simulink model "VehicleSilSimulation"  (R2026a)
settings: configuration reference "standardSILConfigurationParams" (kept outside this file)
StopFcn:
  | fid = fopen('C:\Users\Edison Altamirano\SITLV2\AnelloSummer\optimAeroPX4SIL\HILDiagnostics\logs\session_gtfix1\matlab_error_capture.txt','a'); fprintf(fid, '--- StopFcn fired at %s ---\n', datestr(now)); [m,i] = lasterr(); fprintf(fid, 'lasterr: %s (id: %s)\n', m, i); try; le = lasterror(); fprintf(fid, 'stack:\n'); for k=1:numel(le.stack); fprintf(fid, '  %s line %d\n', le.stack(k).name, le.stack(k).line); end; catch; end; fclose(fid);
values from neighbouring files (symbols this model uses):
  CONTROLLER_RUNTIME = 1    [initVehicleSIL.m]
  stepSize_s = 0.004    [initVehicleSIL.m]
  vehicleParams = evalin('base', 'vehicleParams')    [testVehicleSIL.m]
undefined symbols (not defined in the file or in its folder): actuatorDelay_s, controllerArmed, EngineCommandBus, gpsFreq, heartbeatFreq, opts, Payload, plantSampleTime_s, referenceLatitude_deg, referenceLongitude_deg, SampleTime, ServosCommandBus
libraries: uavmavlinklib x8, simulink x8, instrumentlib x6, flightGearInterfaceLibrary x6, aerolibfltsims x3, sharedtransform x3, px4MAVLinkBridgelib x2, aerolibanimutils x1, hdlsllib x1, dspnetwork x1, robotcorelib x1, uavutilslib x1
(part 3 of 3)

== matlab function VehicleSilSimulation/vehicleSimulation/plant/f22JSBSim/packF22JSBSimInputs ==
  data: posAileron_rad input; jsbsimInputs output; posElevator_rad input; posRudder_rad input; cmdThrottle_unit input; simTime_s input; isVehicleAirborne input; controllerArmed input
function jsbsimInputs = packF22JSBSimInputs(posAileron_rad, posElevator_rad, posRudder_rad, cmdThrottle_unit, simTime_s, isVehicleAirborne, controllerArmed)
%#codegen
% Re-normalizes actuatorsF22JSBSim.slx's achieved (rate-limited) surface positions back to
% JSBSim's fcs/*-cmd-norm convention, using the same real deflection limits as
% setUpActuators.m's "f22jsbsim" case (sourced from f22.xml <flight_control> aerosurface_scale
% ranges: aileron +-0.436 rad/24.98 deg, elevator +-0.5236 rad/30 deg, rudder +-0.5236 rad/30 deg
% -- confirmed by direct grep of aircraft/f22/f22.xml's "Lateral"/"Pitch" channels, see
% PLAN_JSBSIM_SFUNCTION_F22_C130.md Phase A). Throttle is broadcast to both F119-PW-100 engine
% indices -- PX4's MAV_TYPE 1 airframe has only one throttle channel, no independent per-engine
% control in this pass. Output order matches f22JSBSim_io.xml <input> order exactly: aileron,
% elevator, rudder, throttle (bare, engine 0), throttle[1] (engine 1), gear-cmd-norm,
% left-brake-cmd-norm, right-brake-cmd-norm -- do not reorder without updating that file.
%
% PARKING BRAKE / GROUND-ROLL INTERLOCK (added 2026-08-01, PLAN_JSBSIM_SFUNCTION_F22_C130.md
% section 17): f22run-guarded (session_gtfix1) found the plant rolling and accelerating
% completely unsupervised for the ENTIRE ~178s PX4 spends on EKF-alignment/arm retries before
% this vehicle's first "armed" event -- idle turbine thrust (~1300 lbf/engine once the engine-IC
% transient below settles) with no brake command ever wired and only rolling_friction=0.02 lets
% the aircraft reach 32+ m/s before PX4 ever takes control, which is what actually corrupted the
% land-detector/TECS/runway-takeoff state machine downstream (not a sensor bug, not a JSBSim aero
% bug). Fix: hold full parking brake (both fcs/left-brake-cmd-norm and fcs/right-brake-cmd-norm
% at 1.0) AND force commanded throttle to 0 (a second, independent interlock -- this does not
% eliminate turbine idle thrust by itself, brakes carry that load) whenever controllerArmed is
% false. controllerArmed is threaded in from PX4 Interface's own existing (previously
% subsystem-local) "controllerArmed" Goto tag, now exposed as a real port -- see
% VehicleSilSimulation.slx/PX4 Interface and the plant/vehicleSimulation port chain.
%
% RELEASE CONDITION: PX4 Interface does not expose vehicle_status.nav_state or
% vehicle_attitude_setpoint over the HIL link this SIL uses (pixhawk_sil_connector is a
% source-unavailable binary S-Function whose output vector carries mapped servo/actuator values,
% not internal PX4 topics) -- true "active mode is takeoff/mission" and "valid takeoff attitude
% setpoint exists" checks from the user's original spec are therefore not directly observable in
% Simulink. Pragmatic, documented substitute: release once controllerArmed is true AND commanded
% throttle (BEFORE this function's own zero-while-disarmed override, i.e. the raw
% cmdThrottle_unit input) exceeds a small threshold -- PX4 only commands real throttle once it is
% actually trying to taxi/take off, so this approximates "a real takeoff/mission setpoint is
% driving the vehicle" using signals that actually exist here. Debounced 0.75s (persistent sample
% counter at this model's Ts, matches stepSize_s=0.004s/250Hz) before brakes actually release, per
% the user's 0.5-1s debounce request.
releaseThrottleThreshold_unit = 0.05;
debounceTime_s = 0.75;
Ts_s = 0.004;
debounceSamples = round(debounceTime_s / Ts_s);

% ONE-WAY LATCH (added after session_gtfix3, PLAN_JSBSIM_SFUNCTION_F22_C130.md section 18):
% gtfix3's LateralDebug log caught the exact mechanism -- without a latch, brakesReleased was
% recomputed fresh every step from releaseConditionCounter, which resets to 0 on the very next
% sample where cmdThrottle_unit dips at/below the threshold (release requires 0.75s sustained,
% but re-engage was a single-sample trip, no debounce in that direction). PX4 cut throttle to
% ~0 right at rotation (t=25.0-25.27s), which snapped full parking brake back on
% (fcs/left-brake-cmd-norm=fcs/right-brake-cmd-norm=1) for t=25.268-27.936s -- spanning the exact
% moment the aircraft actually left the ground (altitude climbing from t~26s onward, gear still
% commanded down). Reapplying full brake torque during that ground/air transition, when left/right
% main gear compression is momentarily asymmetric, injected a differential drag moment that seeded
% the roll/yaw divergence observed starting t=27.0-27.5s (fcs/aileron-cmd-norm and moments/l-aero-
% lbsft both diverging sharply, well before gear/gear-pos-norm even started retracting at t=28.0).
% Plant-only sign test (f22_lateral_probe.xml) had already cleared aileron/rudder sign and
% aero-derivative defects, and gear-pos-norm stayed at 1.000 through the divergence onset in both
% this run and the earlier session_gtfix2, ruling out the gear-retraction kinematic snap itself as
% the trigger -- it's specifically the brake re-engagement. Fix: once brakes have legitimately
% released (throttle sustained above threshold for the full debounce while armed), never re-engage
% for the rest of the flight -- same one-way latch pattern as gearRetracted below. A real parking
% brake wouldn't be stomped back on mid-rotation just because throttle blipped low for a moment.
persistent releaseConditionCounter brakesEverReleased
if isempty(releaseConditionCounter)
    releaseConditionCounter = int32(0);
end
if isempty(brakesEverReleased)
    brakesEverReleased = false;
end
releaseConditionNow = controllerArmed && (cmdThrottle_unit > releaseThrottleThreshold_unit);
if releaseConditionNow
    releaseConditionCounter = min(releaseConditionCounter + 1, debounceSamples);
else
    releaseConditionCounter = int32(0);
end
if ~brakesEverReleased && releaseConditionCounter >= debounceSamples
    brakesEverReleased = true;
end
brakesReleased = brakesEverReleased;

if ~controllerArmed
    cmdThrottle_unit = 0;
end
%
% gear-cmd-norm retracts once BOTH isVehicleAirborne (Memory-delayed h-agl-ft feedback from
% unpackF22JSBSimOutputs.m) is true AND simTime_s (Clock feedback) exceeds a 5s safety floor -- see
% PLAN_JSBSIM_SFUNCTION_F22_C130.md section 12 for the full history of why this specific condition
% was chosen; short version: f22.xml's "Pitch" channel has a "fcs/gear-down-q-limit" switch that
% caps commanded pitch-rate authority to 30% of normal while gear/gear-pos-norm > 0, and this
% airframe is documented as "10% unstable at subsonic" -- 30% authority alone was confirmed
% (f22run9: softened PX4 demand gains, gear permanently down, NO transition at all) to be
% insufficient for genuine STABILITY, not merely a demand/tracking mismatch -- the aircraft
% diverged into the same uncontrolled nose-up pitch runaway regardless of how gently PX4 asked for
% pitch rate. This rules out "PX4 demanding too much" as the sole cause and means gear MUST
% eventually retract to reach the full authority this airframe's own FCS was designed around.
% Earlier attempts at retraction alone (f22run6/f22run7/f22run8) each hit a different problem
% (spurious premature retraction at t=0; retraction while still parked/unarmed; a violent
% integrator-windup-release snap at the 30%->100% step transition after 22+ seconds of
% authority-limited flight) -- this version combines dynamic retraction with the SAME softened
% FW_P_RMAX_POS/FW_T_CLMB_R_SP/FW_P_LIM_MAX demand gains from the f22run9 attempt, so that
% whatever time is spent in the 30%-limited regime before liftoff accumulates much less
% integrator windup than the original unsoftened gains did, minimizing the severity of the
% eventual authority-restoration transition rather than eliminating the need for it.
%
% gearRetracted LATCH (added after f22run10): isVehicleAirborne is a raw instantaneous h-agl-ft>0.1m
% threshold (see unpackF22JSBSimOutputs.m), only delayed by a single step through the Memory block --
% NOT debounced. f22run10's groundtruth (vehicle_local_position_groundtruth in the resulting .ulg)
% showed the aircraft sitting still until simTime_s crossed 5s, then bouncing violently (z
% oscillating ~0.7-1.6m, vz swinging +-3 m/s) for ~17s before finally launching uncontrolled -- the
% bounce onset lines up exactly with the 5s floor arming the retract condition. Root cause: with
% zero gear-traverse-time (the same C130 lesson applied proactively in f22.xml), any ground-contact
% bounce that nudges h-agl-ft back and forth across the 0.1m threshold makes isVehicleAirborne (and
% therefore gearCmd_norm) chatter every step; gear position then snaps instantly on every chatter,
% injecting a contact-force impulse each time -- a resonant feedback loop that eventually threw the
% aircraft airborne rather than letting it settle. Fix: gear retraction is now a one-way persistent
% latch -- once the airborne+5s condition is true for a single step, gearRetracted stays true.
% A separate landing-extension latch below may subsequently command the gear down, but never lets
% it chatter back up after touchdown. This eliminates the takeoff chatter without
% reintroducing either of the f22run6/f22run7 premature-retraction regressions, since the latch only
% ever transitions 0->1, never back.
maxAilDefl_rad = 0.436;
maxElevatorDefl_rad = 0.5236;
maxRudderDefl_rad = 0.5236;

aileronCmd_norm = max(min(posAileron_rad / maxAilDefl_rad, 1), -1);
elevatorCmd_norm = max(min(posElevator_rad / maxElevatorDefl_rad, 1), -1);
rudderCmd_norm = max(min(posRudder_rad / maxRudderDefl_rad, 1), -1);
throttleCmd_norm = max(min(cmdThrottle_unit, 1), 0);

persistent gearRetracted gearExtendedForLanding
if isempty(gearRetracted)
    gearRetracted = false;
end
if isempty(gearExtendedForLanding)
    gearExtendedForLanding = false;
end
if ~gearRetracted && isVehicleAirborne && simTime_s > 5
    gearRetracted = true;
end
% Once a real flight has retracted the gear, the next low-AGL/contact
% indication is the only unambiguous landing cue available through this SIL
% interface. Latch the gear down at that point. The F-22 JSBSim gear has
% zero traverse time, so restoring contact geometry on this first sample
% prevents the aircraft from falling through the terrain during RTL. The
% latch also prevents the old gear chatter if the aircraft bounces.
if gearRetracted && ~gearExtendedForLanding && ~isVehicleAirborne
    gearExtendedForLanding = true;
end
gearCmd_norm = double(~gearRetracted || gearExtendedForLanding);

% Reapply symmetric wheel braking only after the landing-extension latch has
% observed the first post-flight ground contact.  brakesEverReleased must
% remain one-way during takeoff (see above), but leaving both brakes at zero
% forever made the F-22 roll/bounce beyond the 1000 s mission horizon after a
% valid NAV_LAND touchdown.  The landing latch is unavailable until the gear
% has first retracted in real flight, so this cannot reintroduce parking-brake
% chatter during rotation.  Symmetric commands also avoid a yaw impulse.
landingBrakeApplied = gearExtendedForLanding;
if ~brakesReleased || landingBrakeApplied
    leftBrakeCmd_norm = 1;
    rightBrakeCmd_norm = 1;
else
    leftBrakeCmd_norm = 0;
    rightBrakeCmd_norm = 0;
end

jsbsimInputs = [aileronCmd_norm; elevatorCmd_norm; rudderCmd_norm; ...
                throttleCmd_norm; throttleCmd_norm; ...
                gearCmd_norm; leftBrakeCmd_norm; rightBrakeCmd_norm];
end

== matlab function VehicleSilSimulation/vehicleSimulation/plant/f22JSBSim/unpackF22JSBSimOutputs ==
  data: jsbsimState input; aircraftVelInNED_mps output; jsbsimAero input; gravityScalar_mps2 input; referenceLatitude_deg input; referenceLongitude_deg input; aircraftPosInNED_m output; aircraftEulerAngles_rad output; aircraftVelInBody_mps output; aircraftAngVelInBody_radps output; aircraftAngAccelInBody_radps2 output; aircraftAccelInBody_mps2 output; DCM_be output; aircraftAccelbe_mps2 output; airspeedInBody_mps output; alpha_rad output; beta_rad output; isVehicleAirborne output
function [aircraftVelInNED_mps, aircraftPosInNED_m, aircraftEulerAngles_rad, ...
          aircraftVelInBody_mps, aircraftAngVelInBody_radps, aircraftAngAccelInBody_radps2, ...
          aircraftAccelInBody_mps2, DCM_be, aircraftAccelbe_mps2, ...
          airspeedInBody_mps, alpha_rad, beta_rad, isVehicleAirborne] = ...
          unpackF22JSBSimOutputs(jsbsimState, jsbsimAero, gravityScalar_mps2, ...
          referenceLatitude_deg, referenceLongitude_deg) %#codegen
% Converts JSBSim_SFunction's raw English-unit "State"/"Aero" output vectors (see
% f22JSBSim_io.xml for the exact property order this function assumes) into the SI
% BodyStateBus/AirDataBus fields the rest of this SIL expects. Same conversions as
% c172pJSBSim's/c130JSBSim's own unpack*JSBSimOutputs.m (aircraft-independent physics -- see
% PLAN_JSBSIM_SFUNCTION_HYBRID_C172P.md §2 for the original derivation of each one); only the
% function/file name differs per PLAN_JSBSIM_SFUNCTION_F22_C130.md Phase C.
%
% jsbsimState order (19): lat-gc-deg, long-gc-deg, h-sl-ft, phi-rad, theta-rad, psi-rad, u-fps,
%   v-fps, w-fps, p-rad_sec, q-rad_sec, r-rad_sec, udot-ft_sec2, vdot-ft_sec2, wdot-ft_sec2,
%   pdot-rad_sec2, qdot-rad_sec2, rdot-rad_sec2, h-agl-ft
% jsbsimAero order (5): alpha-rad, beta-rad, u-aero-fps, v-aero-fps, w-aero-fps
ft2m = 0.3048;

lat_deg     = jsbsimState(1);
lon_deg     = jsbsimState(2);
h_sl_ft     = jsbsimState(3);
phi_rad     = jsbsimState(4);
theta_rad   = jsbsimState(5);
psi_rad     = jsbsimState(6);
u_fps       = jsbsimState(7);
v_fps       = jsbsimState(8);
w_fps       = jsbsimState(9);
p_radps     = jsbsimState(10);
q_radps     = jsbsimState(11);
r_radps     = jsbsimState(12);
udot_ftps2  = jsbsimState(13);
vdot_ftps2  = jsbsimState(14);
wdot_ftps2  = jsbsimState(15);
pdot_radps2 = jsbsimState(16);
qdot_radps2 = jsbsimState(17);
rdot_radps2 = jsbsimState(18);
h_agl_ft    = jsbsimState(19);

alpha_rad = jsbsimAero(1);
beta_rad  = jsbsimAero(2);
u_aero_fps = jsbsimAero(3);
v_aero_fps = jsbsimAero(4);
w_aero_fps = jsbsimAero(5);

% Nav (NED) -> body DCM, standard 3-2-1 Euler sequence (Aerospace Toolbox, codegen-compatible).
DCM_be = angle2dcm(psi_rad, theta_rad, phi_rad);

% Local flat-Earth tangent-plane position, anchored at this vehicle's own reference lat/lon (same
% point setUpVehicle.m's "f22jsbsim" case and f22JSBSimInit.xml use), with zDown absolute
% (-h_sl_ft*ft2m), matching every other vehicle's aircraftInitialPosInNED_m convention. Hand-coded
% spherical equirectangular approximation instead of Aerospace Toolbox's lla2flat -- lla2flat
% breaks Simulink's MATLAB Function block type inference in this MATLAB release (confirmed by
% isolated reproduction during c172pJSBSim's own Phase C, same bug class documented in
% optimAeroPX4SIL/CLAUDE.md section 3). At the sub-100km scale this SIL operates at, the
% spherical/WGS84 difference is negligible.
earthRadius_m = 6371000;
dLat_rad = (lat_deg - referenceLatitude_deg) * pi/180;
dLon_rad = (lon_deg - referenceLongitude_deg) * pi/180;
xNorth_m = dLat_rad * earthRadius_m;
yEast_m = dLon_rad * earthRadius_m * cos(referenceLatitude_deg * pi/180);
zDown_m = -h_sl_ft * ft2m;
aircraftPosInNED_m = [xNorth_m; yEast_m; zDown_m];

aircraftVelInBody_mps = [u_fps; v_fps; w_fps] * ft2m;
aircraftVelInNED_mps = DCM_be' * aircraftVelInBody_mps;

aircraftAngVelInBody_radps = [p_radps; q_radps; r_radps];
aircraftAngAccelInBody_radps2 = [pdot_radps2; qdot_radps2; rdot_radps2];

% JSBSim's accelerations/{u,v,w}dot-ft_sec2 are TOTAL body-axis acceleration at the CG (includes
% gravity's contribution via the equations of motion) -- i.e. the same "raw inertial acceleration"
% quantity every other vehicle's plant supplies for this field. `aircraftAccelbe_mps2` must stay
% the RAW acceleration here, NOT specific force: both ins.slx's "Three-axis Inertial Measurement
% Unit" block (aerolibnav) and ANELLO_X3_IMU_Vehicle_fcn_SIL.m already subtract gravity themselves
% (their own g_body/Gb input) to turn raw acceleration into specific force. Subtracting gravity a
% second time here would double-count it. This is also why no gravity_body term appears below --
% "raw inertial acceleration" (accelInertial_body) IS this function's contract, not specific force;
% subtracting gravity here would violate that contract and double-count it downstream, exactly the
% failure mode the comment above already warns about.
%
% CENTRIPETAL/CORIOLIS CORRECTION (2026-08-01, ported from the c130JSBSim fix -- see
% PLAN_JSBSIM_SFUNCTION_F22_C130.md section 14.1/15 for the full derivation and c130JSBSim's own
% confirmed-working live-test evidence): udot/vdot/wdot as JSBSim computes them (FGPropagate:
% vUVWdot = vForces/mass - vPQR x vUVW) are the component-wise derivative of the body velocity
% vector AS SEEN IN THE ROTATING BODY FRAME (dV/dt|_body) -- NOT the true inertial acceleration
% expressed in body axes. By the rotating-frame transport theorem (Stevens & Lewis "Aircraft
% Control and Simulation"):
%   accelInertial_body = dV/dt|_body + omega_body x velocity_body
% Convert velocity and its derivative to SI FIRST, then take the cross product (omega_body is
% already rad/s, dimensionless x 1/time, no conversion needed) -- this is a first-principles
% physics bug independent of any particular airframe, confirmed and fixed for c130JSBSim first;
% same missing term here. Applying it before attributing F-22's own pitch-runaway divergence to
% aero data (aero/coefficient/Cmalpha/Cmq, PLAN_JSBSIM_SFUNCTION_F22_C130.md section 13.6) --
% that divergence was isolated via Simulink's own JSBSim-groundtruth state (not an EKF/estimator
% artifact), so this fix is not expected to eliminate it by itself, but it changes what the
% simulated accelerometer feeds to PX4's own attitude/rate estimator during rotation, which can
% feed back into the real control response -- must be ruled out before concluding aero-table work
% is the only remaining lever.
omega_body_radps = [p_radps; q_radps; r_radps];
velocity_body_mps = [u_fps; v_fps; w_fps] * ft2m;
accelBodyFrame_mps2 = [udot_ftps2; vdot_ftps2; wdot_ftps2] * ft2m;
omegaCrossV_mps2 = [omega_body_radps(2)*velocity_body_mps(3) - omega_body_radps(3)*velocity_body_mps(2); ...
                    omega_body_radps(3)*velocity_body_mps(1) - omega_body_radps(1)*velocity_body_mps(3); ...
                    omega_body_radps(1)*velocity_body_mps(2) - omega_body_radps(2)*velocity_body_mps(1)];
aircraftAccelInBody_mps2 = accelBodyFrame_mps2 + omegaCrossV_mps2;
aircraftAccelbe_mps2 = aircraftAccelInBody_mps2;

aircraftEulerAngles_rad = [phi_rad; theta_rad; psi_rad];

% Airmass-relative body-axis velocity (wind-inclusive) for AirDataBus -- NOT the inertial u/v/w.
airspeedInBody_mps = [u_aero_fps; v_aero_fps; w_aero_fps] * ft2m;

% Threshold intentionally much higher than C130's/C172p's 0.1m convention -- f22JSBSimInit.xml's
% corrected IC altitude means F-22 sits ~5.5ft (1.68m) AGL at rest on its own extended gear (a real
% geometry fact, confirmed by a standalone plant settle test: 5.44-5.56ft), so a 0.1m threshold is
% ALWAYS true even parked, unarmed, on the runway. f22run13's groundtruth (vehicle_local_position_
% groundtruth) showed this directly: the one-way gearRetracted latch in packF22JSBSimInputs.m fired
% the instant simTime_s crossed 5s (isVehicleAirborne having been spuriously true from t=0), and the
% still-parked, still-disarmed aircraft free-fell at a clean 9.8 m/s^2 once its gear support was
% pulled out from under it. 15ft/4.572m is comfortably above the ~5.5ft at-rest height (with margin
% for gear-compression settling noise) while still being low enough to trip promptly once genuinely
% climbing out after a real takeoff.
isVehicleAirborne = (h_agl_ft * ft2m) > 4.572;
end

== matlab function VehicleSilSimulation/F22AbortCheck ==
  data: angVel input; abortFlag output; euler input; isF22Active input
function abortFlag = f22AbortCheck(angVel, euler, isF22Active)
%#codegen
% p/q threshold set to 1.5 rad/s (2026-08-02, PLAN_JSBSIM_SFUNCTION_F22_C130.md section 18):
% the original 0.8 rad/s gate was tripping on a legitimate, bounded rotation-transient roll
% settle, confirmed via gtfix7diag (a one-off diagnostic run with this threshold temporarily
% widened to 3.0): p peaked at ~0.87 rad/s while the aircraft settled into a stable, if
% oversized, ~45deg bank rather than diverging further -- the mission then completed takeoff,
% climb to target altitude/airspeed, the guarded waypoint, and RTL handoff with no crash.
% 1.5 rad/s keeps real margin above that confirmed-benign peak while still catching genuine
% divergence (prior crashes reached 0.80 within ~0.3-0.5s of onset and kept accelerating,
% unlike this bounded case). The ~45deg bank-hold itself is a separate, still-open issue
% (residual lateral trim/control error, not a crash risk) tracked apart from this gate.
p = angVel(1);
q = angVel(2);
pitchRad = euler(2);
abortFlag = isF22Active && (abs(p) > 1.5 || abs(q) > 1.5 || abs(pitchRad) > 60*pi/180);
end

== matlab function VehicleSilSimulation/vehicleSimulation/plant/c172pJSBSim/packJSBSimInputs ==
  data: posAileron_rad input; jsbsimInputs output; posElevator_rad input; posRudder_rad input; cmdThrottle_unit input
function jsbsimInputs = packJSBSimInputs(posAileron_rad, posElevator_rad, posRudder_rad, cmdThrottle_unit)
%#codegen
% Re-normalizes actuatorsC172p.slx's achieved (rate-limited) surface positions back to JSBSim's
% fcs/*-cmd-norm convention, using the same real deflection limits as setUpActuators.m's "c172p"
% case (sourced from c172p.xml <flight_control> aerosurface_scale ranges: elevator 28 deg,
% aileron 20 deg, rudder 16 deg). Throttle is passed straight through (already 0..1 normalized,
% not rate-limited by actuatorsC172p). Output order matches c172pJSBSim_io.xml <input> order
% exactly: aileron, elevator, rudder, throttle -- do not reorder without updating that file.
maxAilDefl_rad = 20 * pi/180;
maxElevatorDefl_rad = 28 * pi/180;
maxRudderDefl_rad = 16 * pi/180;

aileronCmd_norm = max(min(posAileron_rad / maxAilDefl_rad, 1), -1);
elevatorCmd_norm = max(min(posElevator_rad / maxElevatorDefl_rad, 1), -1);
rudderCmd_norm = max(min(posRudder_rad / maxRudderDefl_rad, 1), -1);
throttleCmd_norm = max(min(cmdThrottle_unit, 1), 0);

jsbsimInputs = [aileronCmd_norm; elevatorCmd_norm; rudderCmd_norm; throttleCmd_norm];
end

== matlab function VehicleSilSimulation/CheckAbort ==
  data: angVel input; abortFlag output; pos input; velNED input; euler input
function abortFlag = checkAbort(angVel, pos, velNED, euler)
%#codegen
% Speed threshold raised 80->200 m/s and roll/pitch thresholds raised 60->85 deg
% (2026-08-01, PLAN_JSBSIM_SFUNCTION_F22_C130.md section 11/12): this check exists to catch
% genuine numerical divergence (NaN/Inf, runaway blow-ups), not to enforce a realistic
% per-vehicle flight envelope. Confirmed via .ulg groundtruth analysis of two separate live
% sessions that this block was the actual cause of two previously-unexplained mid-flight
% simulation stops: f22JSBSim's own designed cruise speed (100 m/s trim) exceeded the old
% 80 m/s speed limit (f22run2 stopped at groundspeed=79.3 m/s, still smoothly accelerating,
% no divergence); c130JSBSim's roll angle reached exactly 60.0 deg during a normal waypoint
% turn in c130run6 (confirmed via vehicle_attitude_groundtruth quaternion analysis, roll
% climbing smoothly from ~37deg over the prior several seconds, not oscillating/diverging) and
% the sim stopped in the same instant. Both are false positives from this shared,
% vehicle-agnostic safety net -- not real vehicle bugs. 200 m/s and 85 deg are comfortably
% above both vehicles' real operating envelopes while still catching true numerical blow-ups
% (this SIL's own history has produced groundspeeds/attitudes far beyond these bounds during
% genuine divergence, e.g. the pre-fix c130JSBSim engine-torque bug).
speed = sqrt(sum(velNED.^2));
rollDeg = abs(euler(1))*180/pi;
pitchDeg = abs(euler(2))*180/pi;
bodyRateNorm = sqrt(sum(angVel.^2));
badPos = any(~isfinite(pos)) || pos(3) > 15 || pos(3) < -600;
abortFlag = (speed > 200) || (rollDeg > 85) || (pitchDeg > 85) || (bodyRateNorm > 3) || badPos || any(~isfinite(velNED)) || any(~isfinite(euler));
end

== matlab function VehicleSilSimulation/vehicleSimulation/plant/c130JSBSim/packC130JSBSimInputs ==
  data: posAileron_rad input; jsbsimInputs output; posElevator_rad input; posRudder_rad input; cmdThrottle_unit input
function jsbsimInputs = packC130JSBSimInputs(posAileron_rad, posElevator_rad, posRudder_rad, cmdThrottle_unit)
%#codegen
% Re-normalizes actuatorsC130JSBSim.slx's achieved (rate-limited) surface positions back to
% JSBSim's fcs/*-cmd-norm convention, using the same real deflection limits as
% setUpActuators.m's "c130jsbsim" case (sourced from C130.xml <flight_control> aerosurface_scale
% ranges: elevator -0.35/+0.3 rad, aileron/rudder +-0.35 rad -- symmetric +-0.35 rad/20.05 deg used
% here for all three, same "store/use the larger magnitude" convention as setUpActuators.m).
% Throttle is broadcast to all 4 T56 engine indices -- PX4's MAV_TYPE 1 airframe has only one
% throttle channel, no independent per-engine control in this pass (see
% PLAN_JSBSIM_SFUNCTION_F22_C130.md Phase B). Output order matches c130JSBSim_io.xml <input> order
% exactly: aileron, elevator, rudder, throttle[0], throttle[1], throttle[2], throttle[3],
% gear-cmd-norm, left brake, right brake -- do not reorder without updating that file.
% gear-cmd-norm is a hardcoded 1.0
% (gear permanently down, never retracts) -- see c130JSBSim_io.xml's header comment for why this
% is required (unlike c172p's fixed gear, C130's gear is retractable and defaults to 0/up if left
% undriven, which would remove ground-contact support entirely at simulation start).
maxAilDefl_rad = 20.05 * pi/180;
maxElevatorDefl_rad = 20.05 * pi/180;
maxRudderDefl_rad = 20.05 * pi/180;

aileronCmd_norm = max(min(posAileron_rad / maxAilDefl_rad, 1), -1);
elevatorCmd_norm = max(min(posElevator_rad / maxElevatorDefl_rad, 1), -1);
rudderCmd_norm = max(min(posRudder_rad / maxRudderDefl_rad, 1), -1);
throttleCmd_norm = max(min(cmdThrottle_unit, 1), 0);
gearCmd_norm = 1;
% Running T56 engines produce enough idle thrust to move the aircraft while
% PX4/MAVSDK are still connecting. Hold both main-wheel brakes at idle and
% release them as soon as PX4 commands meaningful takeoff power. Reapplying
% this rule after touchdown also lets PX4 confirm landed/disarmed.
brakeCmd_norm = double(throttleCmd_norm < 0.05);

jsbsimInputs = [aileronCmd_norm; elevatorCmd_norm; rudderCmd_norm; ...
                throttleCmd_norm; throttleCmd_norm; throttleCmd_norm; throttleCmd_norm; ...
                gearCmd_norm; brakeCmd_norm; brakeCmd_norm];
end

== matlab function VehicleSilSimulation/vehicleSimulation/plant/c130JSBSim/unpackC130JSBSimOutputs ==
  data: jsbsimState input; aircraftVelInNED_mps output; jsbsimAero input; gravityScalar_mps2 input; referenceLatitude_deg input; referenceLongitude_deg input; aircraftPosInNED_m output; aircraftEulerAngles_rad output; aircraftVelInBody_mps output; aircraftAngVelInBody_radps output; aircraftAngAccelInBody_radps2 output; aircraftAccelInBody_mps2 output; DCM_be output; aircraftAccelbe_mps2 output; airspeedInBody_mps output; alpha_rad output; beta_rad output; isVehicleAirborne output
function [aircraftVelInNED_mps, aircraftPosInNED_m, aircraftEulerAngles_rad, ...
          aircraftVelInBody_mps, aircraftAngVelInBody_radps, aircraftAngAccelInBody_radps2, ...
          aircraftAccelInBody_mps2, DCM_be, aircraftAccelbe_mps2, ...
          airspeedInBody_mps, alpha_rad, beta_rad, isVehicleAirborne] = ...
          unpackC130JSBSimOutputs(jsbsimState, jsbsimAero, gravityScalar_mps2, ...
          referenceLatitude_deg, referenceLongitude_deg) %#codegen
% Converts JSBSim_SFunction's raw English-unit "State"/"Aero" output vectors (see
% c130JSBSim_io.xml for the exact property order this function assumes) into the SI
% BodyStateBus/AirDataBus fields the rest of this SIL expects. Same conversions as
% c172pJSBSim's own unpackJSBSimOutputs.m (aircraft-independent physics -- see
% PLAN_JSBSIM_SFUNCTION_HYBRID_C172P.md §2 for the original derivation of each one); only the
% function/file name differs per PLAN_JSBSIM_SFUNCTION_F22_C130.md Phase C.
%
% jsbsimState order (19): lat-gc-deg, long-gc-deg, h-sl-ft, phi-rad, theta-rad, psi-rad, u-fps,
%   v-fps, w-fps, p-rad_sec, q-rad_sec, r-rad_sec, udot-ft_sec2, vdot-ft_sec2, wdot-ft_sec2,
%   pdot-rad_sec2, qdot-rad_sec2, rdot-rad_sec2, h-agl-ft
% jsbsimAero order (5): alpha-rad, beta-rad, u-aero-fps, v-aero-fps, w-aero-fps
ft2m = 0.3048;

lat_deg     = jsbsimState(1);
lon_deg     = jsbsimState(2);
h_sl_ft     = jsbsimState(3);
phi_rad     = jsbsimState(4);
theta_rad   = jsbsimState(5);
psi_rad     = jsbsimState(6);
u_fps       = jsbsimState(7);
v_fps       = jsbsimState(8);
w_fps       = jsbsimState(9);
p_radps     = jsbsimState(10);
q_radps     = jsbsimState(11);
r_radps     = jsbsimState(12);
udot_ftps2  = jsbsimState(13);
vdot_ftps2  = jsbsimState(14);
wdot_ftps2  = jsbsimState(15);
pdot_radps2 = jsbsimState(16);
qdot_radps2 = jsbsimState(17);
rdot_radps2 = jsbsimState(18);
h_agl_ft    = jsbsimState(19);

alpha_rad = jsbsimAero(1);
beta_rad  = jsbsimAero(2);
u_aero_fps = jsbsimAero(3);
v_aero_fps = jsbsimAero(4);
w_aero_fps = jsbsimAero(5);

% Nav (NED) -> body DCM, standard 3-2-1 Euler sequence (Aerospace Toolbox, codegen-compatible).
DCM_be = angle2dcm(psi_rad, theta_rad, phi_rad);

% Local flat-Earth tangent-plane position, anchored at this vehicle's own reference lat/lon (same
% point setUpVehicle.m's "c130jsbsim" case and c130JSBSimInit.xml use), with zDown absolute
% (-h_sl_ft*ft2m), matching every other vehicle's aircraftInitialPosInNED_m convention. Hand-coded
% spherical equirectangular approximation instead of Aerospace Toolbox's lla2flat -- lla2flat
% breaks Simulink's MATLAB Function block type inference in this MATLAB release (confirmed by
% isolated reproduction during c172pJSBSim's own Phase C, same bug class documented in
% optimAeroPX4SIL/CLAUDE.md section 3). At the sub-100km scale this SIL operates at, the
% spherical/WGS84 difference is negligible.
earthRadius_m = 6371000;
dLat_rad = (lat_deg - referenceLatitude_deg) * pi/180;
dLon_rad = (lon_deg - referenceLongitude_deg) * pi/180;
xNorth_m = dLat_rad * earthRadius_m;
yEast_m = dLon_rad * earthRadius_m * cos(referenceLatitude_deg * pi/180);
zDown_m = -h_sl_ft * ft2m;
aircraftPosInNED_m = [xNorth_m; yEast_m; zDown_m];

aircraftVelInBody_mps = [u_fps; v_fps; w_fps] * ft2m;
aircraftVelInNED_mps = DCM_be' * aircraftVelInBody_mps;

aircraftAngVelInBody_radps = [p_radps; q_radps; r_radps];
aircraftAngAccelInBody_radps2 = [pdot_radps2; qdot_radps2; rdot_radps2];

% JSBSim's accelerations/{u,v,w}dot-ft_sec2 are TOTAL body-axis acceleration at the CG (includes
% gravity's contribution via the equations of motion) -- i.e. the same "raw inertial acceleration"
% quantity every other vehicle's plant supplies for this field. `aircraftAccelbe_mps2` must stay
% the RAW acceleration here, NOT specific force: both ins.slx's "Three-axis Inertial Measurement
% Unit" block (aerolibnav) and ANELLO_X3_IMU_Vehicle_fcn_SIL.m already subtract gravity themselves
% (their own g_body/Gb input) to turn raw acceleration into specific force. Subtracting gravity a
% second time here would double-count it.
%
% CENTRIPETAL/CORIOLIS CORRECTION (2026-08-01, c130run7/8 post-mortem,
% PLAN_JSBSIM_SFUNCTION_F22_C130.md section 13.9): udot/vdot/wdot as JSBSim computes them
% (FGPropagate: vUVWdot = vForces/mass - vPQR x vUVW) are the component-wise derivative of the
% body velocity vector AS SEEN IN THE ROTATING BODY FRAME (dV/dt|_body) -- NOT the true inertial
% acceleration expressed in body axes. By the rotating-frame transport theorem (standard flight
% dynamics, e.g. Stevens & Lewis "Aircraft Control and Simulation"):
%   a_inertial_body = dV/dt|_body + omega x V
% Previously the omega x V term was omitted entirely, so the "raw acceleration" fed to every
% downstream accelerometer/IMU model was silently missing this centripetal/Coriolis coupling
% term -- exactly zero during straight, non-rotating flight (which is why this was never caught
% before), but growing with p/q/r during any coordinated turn, i.e. precisely when this SIL's own
% C130 EKF2 divergence was observed. Not yet confirmed as THE root cause (needs re-test), but this
% is a genuine, first-principles-derived correctness bug independent of that investigation.
omegaCrossV_ftps2 = [q_radps*w_fps - r_radps*v_fps; ...
                     r_radps*u_fps - p_radps*w_fps; ...
                     p_radps*v_fps - q_radps*u_fps];
aircraftAccelInBody_mps2 = ([udot_ftps2; vdot_ftps2; wdot_ftps2] + omegaCrossV_ftps2) * ft2m;
aircraftAccelbe_mps2 = aircraftAccelInBody_mps2;

aircraftEulerAngles_rad = [phi_rad; theta_rad; psi_rad];

% Airmass-relative body-axis velocity (wind-inclusive) for AirDataBus -- NOT the inertial u/v/w.
airspeedInBody_mps = [u_aero_fps; v_aero_fps; w_aero_fps] * ft2m;

isVehicleAirborne = (h_agl_ft * ft2m) > 0.1;
end

== matlab function VehicleSilSimulation/vehicleSimulation/plant/c172pJSBSim/unpackJSBSimOutputs ==
  data: jsbsimState input size=19; aircraftVelInNED_mps output size=3; jsbsimAero input size=5; gravityScalar_mps2 input size=1; referenceLatitude_deg input size=1; referenceLongitude_deg input size=1; aircraftPosInNED_m output size=3; aircraftEulerAngles_rad output size=3; aircraftVelInBody_mps output size=3; aircraftAngVelInBody_radps output size=3; aircraftAngAccelInBody_radps2 output size=3; aircraftAccelInBody_mps2 output size=3; DCM_be output size=[3 3]; aircraftAccelbe_mps2 output size=3; airspeedInBody_mps output size=3; alpha_rad output size=1; beta_rad output size=1; isVehicleAirborne output size=1
function [aircraftVelInNED_mps, aircraftPosInNED_m, aircraftEulerAngles_rad, ...
          aircraftVelInBody_mps, aircraftAngVelInBody_radps, aircraftAngAccelInBody_radps2, ...
          aircraftAccelInBody_mps2, DCM_be, aircraftAccelbe_mps2, ...
          airspeedInBody_mps, alpha_rad, beta_rad, isVehicleAirborne] = ...
          unpackJSBSimOutputs(jsbsimState, jsbsimAero, gravityScalar_mps2, ...
          referenceLatitude_deg, referenceLongitude_deg) %#codegen
% Converts JSBSim_SFunction's raw English-unit "State"/"Aero" output vectors (see
% aircraft/c172p/c172pJSBSim_io.xml for the exact property order this function assumes) into the SI
% BodyStateBus/AirDataBus fields the rest of this SIL expects. See
% PLAN_JSBSIM_SFUNCTION_HYBRID_C172P.md Phase B/C for why each conversion was chosen.
%
% jsbsimState order (19): lat-gc-deg, long-gc-deg, h-sl-ft, phi-rad, theta-rad, psi-rad, u-fps,
%   v-fps, w-fps, p-rad_sec, q-rad_sec, r-rad_sec, udot-ft_sec2, vdot-ft_sec2, wdot-ft_sec2,
%   pdot-rad_sec2, qdot-rad_sec2, rdot-rad_sec2, h-agl-ft
% jsbsimAero order (5): alpha-rad, beta-rad, u-aero-fps, v-aero-fps, w-aero-fps
ft2m = 0.3048;

lat_deg     = jsbsimState(1);
lon_deg     = jsbsimState(2);
h_sl_ft     = jsbsimState(3);
phi_rad     = jsbsimState(4);
theta_rad   = jsbsimState(5);
psi_rad     = jsbsimState(6);
u_fps       = jsbsimState(7);
v_fps       = jsbsimState(8);
w_fps       = jsbsimState(9);
p_radps     = jsbsimState(10);
q_radps     = jsbsimState(11);
r_radps     = jsbsimState(12);
udot_ftps2  = jsbsimState(13);
vdot_ftps2  = jsbsimState(14);
wdot_ftps2  = jsbsimState(15);
pdot_radps2 = jsbsimState(16);
qdot_radps2 = jsbsimState(17);
rdot_radps2 = jsbsimState(18);
h_agl_ft    = jsbsimState(19);

alpha_rad = jsbsimAero(1);
beta_rad  = jsbsimAero(2);
u_aero_fps = jsbsimAero(3);
v_aero_fps = jsbsimAero(4);
w_aero_fps = jsbsimAero(5);

% Nav (NED) -> body DCM, standard 3-2-1 Euler sequence (Aerospace Toolbox, codegen-compatible).
DCM_be = angle2dcm(psi_rad, theta_rad, phi_rad);

% Local flat-Earth tangent-plane position, anchored at this vehicle's own reference lat/lon (same
% point setUpVehicle.m's "c172pJSBSim" case and c172pJSBSimInit.xml use), with zDown absolute
% (-h_sl_ft*ft2m), matching every other vehicle's aircraftInitialPosInNED_m convention (NED origin
% at sea level / height 0, not at the reference altitude). Hand-coded spherical equirectangular
% approximation instead of Aerospace Toolbox's lla2flat -- lla2flat breaks Simulink's MATLAB
% Function block type inference in this MATLAB release (confirmed by isolated reproduction; same
% bug class as the one already documented in optimAeroPX4SIL/CLAUDE.md section 3 for a different
% toolbox call). At the sub-100km scale this SIL operates at, the spherical/WGS84 difference is
% negligible and this SIL has no other geodetic-accuracy requirement anywhere else.
earthRadius_m = 6371000;
dLat_rad = (lat_deg - referenceLatitude_deg) * pi/180;
dLon_rad = (lon_deg - referenceLongitude_deg) * pi/180;
xNorth_m = dLat_rad * earthRadius_m;
yEast_m = dLon_rad * earthRadius_m * cos(referenceLatitude_deg * pi/180);
zDown_m = -h_sl_ft * ft2m;
aircraftPosInNED_m = [xNorth_m; yEast_m; zDown_m];

aircraftVelInBody_mps = [u_fps; v_fps; w_fps] * ft2m;
aircraftVelInNED_mps = DCM_be' * aircraftVelInBody_mps;

aircraftAngVelInBody_radps = [p_radps; q_radps; r_radps];
aircraftAngAccelInBody_radps2 = [pdot_radps2; qdot_radps2; rdot_radps2];

% Both INS implementations form specific force downstream as f = Ab - g_body. JSBSim's
% accelerations/{u,v,w}dot are derivatives in the rotating body frame, so convert them to inertial
% acceleration expressed in body axes by adding omega x V. Do not add or subtract gravity here:
% a stationary ground run proves that this transport-corrected value is approximately zero, after
% which the INS correctly reports specific force ~= -g. Adding gravity here produced ~0 g at rest;
% omitting the transport correction in a stale embedded chart produced ~-2 g. This matches the
% validated reliability implementation in commit 05badb3.
%
% udot/vdot/wdot alone is dV/dt as seen in the ROTATING BODY FRAME (JSBSim's FGPropagate: vUVWdot =
% vForces/mass - vPQR x vUVW), not the true inertial acceleration expressed in body axes. By the
% rotating-frame transport theorem, a_inertial_body = dV/dt|_body + omega x V. This term is exactly
% zero in straight, non-rotating flight (why this was never caught by earlier c172pJSBSim
% validation) and grows with p/q/r otherwise -- including during ground handling, where idle thrust
% with no parking-brake model can produce nonzero body rates while still disarmed. Same fix already
% applied to unpackC130JSBSimOutputs.m/unpackF22JSBSimOutputs.m (PLAN_JSBSIM_SFUNCTION_F22_C130.md
% section 14.1/15); c172p was flagged there as still carrying this bug and not yet fixed.
omega_body_radps = [p_radps; q_radps; r_radps];
velocity_body_mps = [u_fps; v_fps; w_fps] * ft2m;
accelBodyFrame_mps2 = [udot_ftps2; vdot_ftps2; wdot_ftps2] * ft2m;
omegaCrossV_mps2 = [omega_body_radps(2)*velocity_body_mps(3) - omega_body_radps(3)*velocity_body_mps(2); ...
                    omega_body_radps(3)*velocity_body_mps(1) - omega_body_radps(1)*velocity_body_mps(3); ...
                    omega_body_radps(1)*velocity_body_mps(2) - omega_body_radps(2)*velocity_body_mps(1)];
aircraftAccelInBody_mps2 = accelBodyFrame_mps2 + omegaCrossV_mps2;
aircraftAccelbe_mps2 = aircraftAccelInBody_mps2;

aircraftEulerAngles_rad = [phi_rad; theta_rad; psi_rad];

% Airmass-relative body-axis velocity (wind-inclusive) for AirDataBus -- NOT the inertial u/v/w.
airspeedInBody_mps = [u_aero_fps; v_aero_fps; w_aero_fps] * ft2m;

isVehicleAirborne = (h_agl_ft * ft2m) > 0.1;
end
